simulink model "DrivetrainHevP4"  (R2020a)
settings: Solver=VariableStepAuto  StartTime=0.0  StopTime=inf  RelTol=1e-3  EnableMultiTasking=on
model workspace (MAT data in the model file):
  Aeff = 0.0314159265359
  Af = 2.46
  Bx = 10
  Cd = 0.25
  Cl = 0.1
  Cpm = 0.1
  Cx = 1.65
  Dx = 1
  Ex = 0.01
  FZMAX = 6570
  FZMIN = 0
  Fc = 500
  FsbF = [-700000 -7000 -700 0 700 7000 700000]
  FsbR = [-700000 -7000 -700 0 700 7000 700000]
  FskF = [-8928.57142857 -178.571428571 0 357.142857143 535.714285714 9285.71428571]
  FskR = [-5357.14285714 -107.142857143 0 214.285714286 321.428571429 5571.42857143]
  G = [0 1 2 3 4 5 6]
  G_o = 1
  Iyy = 3000
  Iyy_Whl = 0.8
  J = 0.01
  J1 = 0.01
  J2 = 0.01
  Jd = 0.01
  Ji = 0.2
  Jin = 0.05
  Jin_Cltch = 0.2
  Jin_Cltch2 = 0.01
  Jout = [0.009 0.01 0.01 0.01 0.01 0.01 0.01]
  Jout_Cltch = 0.01
  Jout_Cltch2 = 0.05
  Jt = 0.01
  Jw1 = 0.01
  Jw2 = 0.01
  K_c = 10000
  Lrel = 0.15
  Mass = 1623
  N = [0.001 4.212 2.637 1.8 1.386 1 0.772]
  NF = 2
  NR = 2
  N_P4 = 4.1
  Ndiff = 3.32
  Ndiff_P4 = 4.1
  Ndisk = 1
  Ndisks = 4
  Pabs = 101325
  Press = 7000000
  Re = 0.327
  Reff = 0.11
  Reff_LSD = 0.2
  Rm = 0.15
  T = 300
  Temp_bpts = [313 358]
  Trq_bpts = [25 50 75 100 150 200 250]
  UNLOADED_RADIUS = 0.336
  VXLOW = 2
  aMy = 0.01
  a_CG = 1.09
  alphaMy = 0
  b = Simulink.Parameter
  b.Value = 400
  b.DataType = 'auto'
  b.Dimensions = [1 1]
  b1 = 100
  b1_g = 0.001
  b2 = 100
  b2_g = 0.001
  bMy = 0
  b_CG = 1.7
  b_J = 0.001
  bd = 0.001
  betaMy = 1
  bi = 0.001
  bin = 0.003
  bin_Cltch = 0.003
  bout = [0.003 0.003 0.003 0.003 0.003 0.003 0.003]
  bout_Cltch = 0.003
  br = 0.001
  bt = 0.001
  bw1 = 0.001
  bw2 = 0.001
  cMy = 0
  disk_abore = 0.05
  domega_o = 0
  dw = [0 10 20 40 60 80 100]
  dzdotsF = [-10 -1 -0.1 0 0.1 1 10]
  dzdotsR = [-10 -1 -0.1 0 0.1 1 10]
  dzsF = [-0.005 -0.0001 0 0.2 0.2001 0.2051]
  dzsR = [-0.005 -0.0001 0 0.2 0.2001 0.2051]
  eta = [0.95 0.95 0.95 0.95 0.95 0.95 0.95]
  eta_diff = 0.98
  eta_tbl = [1 1 1 1 1 1 1 1 1 1 1 1 ... (1078 elements, 7x11x7x2)]
  g = 9.81
  h = 0.5
  k = Simulink.Parameter
  k.Value = 10000
  k.DataType = 'auto'
  k.Dimensions = [1 1]
  k1 = 50000
  k2 = 50000
  kappamax = 1.5
  lam_x = 1
  mu_kinetic = 0.35
  mu_static = 0.45
  muc = [0.16 0.13 0.115 0.11 0.105 0.1025 0.10125]
  muk = 0.4
  mus = 0.45
  num_pads = 2
  omega1_c = 3000
  omega2_c = 3000
  omega_bpts = [500.383141081 749.619781963 1002.67614148 1250.9578527 1499.23956393 1747.52127515 1995.80298637 2501.9157054 2998.47912785 4001.15526933 5003.83141081]
  omega_c = Simulink.Parameter
  omega_c.Value = 500
  omega_c.DataType = 'auto'
  omega_c.Dimensions = [1 1]
  omega_o = 0
  omega_o_J = 0
  omegai_o = 0
  omegain_o = 0
  omegal = 94.2477796077
  omegao = 0
  omegaout_o = 0
  omegat_o = 0
  omegau = 83.7758040957
  omegaw1o = 0
  omegaw2o = 0
  phi = [0 0.5 0.6 0.7 0.8 0.87 0.92 0.94 0.96 0.97]
  philu = 0.85
  press = 234400
  psi = [12.2938 12.8588 13.1452 13.6285 14.6163 16.2675 19.3503 22.1046 29.9986 50]
  q_o = 0
  tauC = 0.6
  tauC_1 = 0.1
  tauC_LSD = 0.01
  tauTC = 0.1
  tau_s = 0.08
  tc = 0.01
  theta_o = 0
  theta_o_Veh = 0
  ts = 0.01
  w1_o = 0
  wc = 10
  win_o = 0
  wout_o = 0
  x_o = 0
  xdot_o = 0
  z_o = -0.35
  zdot_o = 0
  zeta = [2.232 1.5462 1.4058 1.2746 1.1528 1.0732 1.0192 0.9983 0.9983 0.9983]
undefined symbols (not defined in the file): Lock, up
libraries: autolibsharedcoupling x4, autolibpowerinfoutils x4, autolibshared x3, autolibshareddiff x2, autolibutils x2, autolibsharedtransfixedgear x1, autolibtrqconv x1
(part 1 of 3)
settings Model: ModifiedByFormat=The MathWorks, Inc.  SimulationMode=accelerator  PauseTimes=10  OrderedModelArguments=off  Creator=The MathWorks, Inc.  LastModifiedBy=The MathWorks, Inc.
settings SolverCC: DecoupledContinuousIntegration=on
settings DataIOCC: DSMLogging=off  ReturnWorkspaceOutputs=off
settings DebuggingCC: MergeDetectMultiDrivingBlocksExec=none  ArithmeticOperatorsInVariantConditions=warning
settings ModelReferenceCC: PropagateSignalLabelsOutOfModel=off
settings SFSimCC: SimUseLocalCustomCode=off
settings RTWCC: RTWUseLocalCustomCode=off
settings CodeAppCC: StateflowObjectComments=on
settings GRTTargetCC: TargetLangStandard=C89/C90 (ANSI)
settings ConfigComp: CovMetricSettings=dsw  CovHtmlReporting=on  CovSaveCumulativeToWorkspaceVar=on  CovSaveSingleToWorkspaceVar=on  CovShowResultsExplorer=off  CovExternalEMLEnable=off
settings SimscapeCC: SimscapeNormalizeSystem=off  SimscapeNominalValues={1, 'bar'; 1, 'cm^3/s'; 1, 'bar*kg/s'; 1, 'kJ/kg'; 1, 'kW'; }

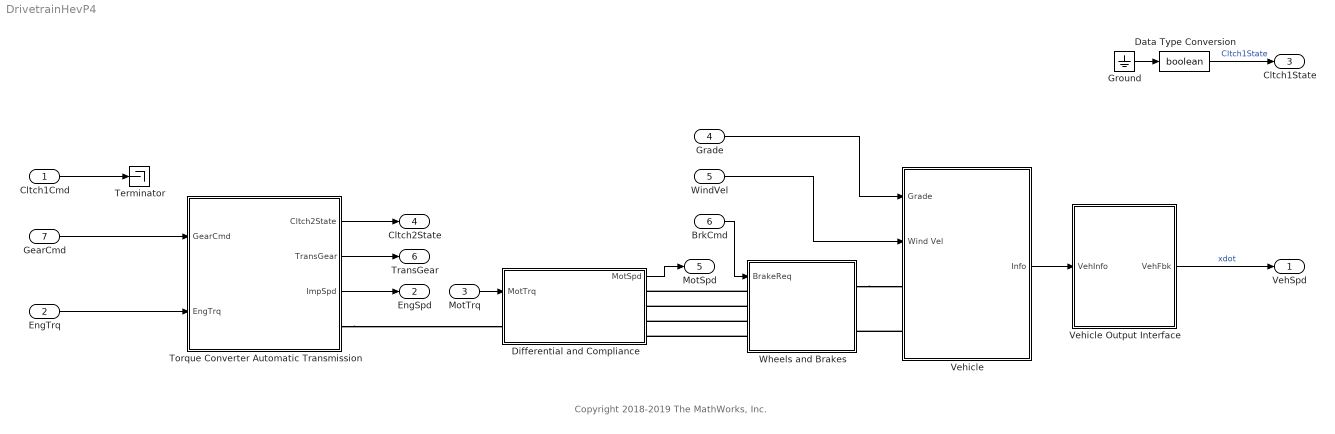
== system DrivetrainHevP4 ==
  note: Copyright 2018-2019 The MathWorks, Inc.
  Cltch1Cmd : Inport
  EngTrq : Inport  Port=2
  MotTrq : Inport  Port=3
  Grade : Inport  Port=4
  WindVel : Inport  Port=5
  BrkCmd : Inport  Port=6
  GearCmd : Inport  Port=7
  Data Type Conversion : DataTypeConversion  OutDataTypeStr=boolean
  Differential and Compliance : Subsystem  VariantControl=2
  Ground : Ground
  Terminator : Terminator
  Torque Converter Automatic Transmission : Subsystem  VariantControl=1
  Vehicle : Subsystem
  Vehicle Output Interface : Subsystem
  Wheels and Brakes : Subsystem  VariantControl=0
  VehSpd : Outport  VectorParamsAs1DForOutWhenUnconnected=off
  EngSpd : Outport  Port=2  VectorParamsAs1DForOutWhenUnconnected=off  BusOutputAsStruct=on
  Cltch1State : Outport  Port=3  VectorParamsAs1DForOutWhenUnconnected=off  BusOutputAsStruct=on
  Cltch2State : Outport  Port=4  VectorParamsAs1DForOutWhenUnconnected=off  BusOutputAsStruct=on
  MotSpd : Outport  Port=5  VectorParamsAs1DForOutWhenUnconnected=off  BusOutputAsStruct=on
  TransGear : Outport  Port=6  VectorParamsAs1DForOutWhenUnconnected=off  BusOutputAsStruct=on
  wires:
  BrkCmd/1 -> Wheels and Brakes/1(BrakeReq)
  Vehicle/1(Info) -> Vehicle Output Interface/1(VehInfo)
  Vehicle Output Interface/1(VehFbk) -> VehSpd/1  "xdot"
  Grade/1 -> Vehicle/1(Grade)
  WindVel/1 -> Vehicle/2(Wind Vel)
  Ground/1 -> Data Type Conversion/1
  Data Type Conversion/1 -> Cltch1State/1  "Cltch1State"
  Torque Converter Automatic Transmission/1(Cltch2State) -> Cltch2State/1
  Torque Converter Automatic Transmission/2(TransGear) -> TransGear/1
  Cltch1Cmd/1 -> Terminator/1
  GearCmd/1 -> Torque Converter Automatic Transmission/1(GearCmd)
  MotTrq/1 -> Differential and Compliance/1(MotTrq)
  EngTrq/1 -> Torque Converter Automatic Transmission/2(EngTrq)
  Torque Converter Automatic Transmission/3(ImpSpd) -> EngSpd/1
  Differential and Compliance/1(MotSpd) -> MotSpd/1
  connections:
  Wheels and Brakes/RConn1 -- Vehicle/LConn1
  Wheels and Brakes/LConn1 -- Differential and Compliance/RConn1
  Wheels and Brakes/LConn3 -- Differential and Compliance/RConn3
  Wheels and Brakes/LConn2 -- Differential and Compliance/RConn2
  Wheels and Brakes/LConn4 -- Differential and Compliance/RConn4
  Vehicle/LConn2 -- Wheels and Brakes/RConn2
  Torque Converter Automatic Transmission/RConn1 -- Differential and Compliance/LConn1

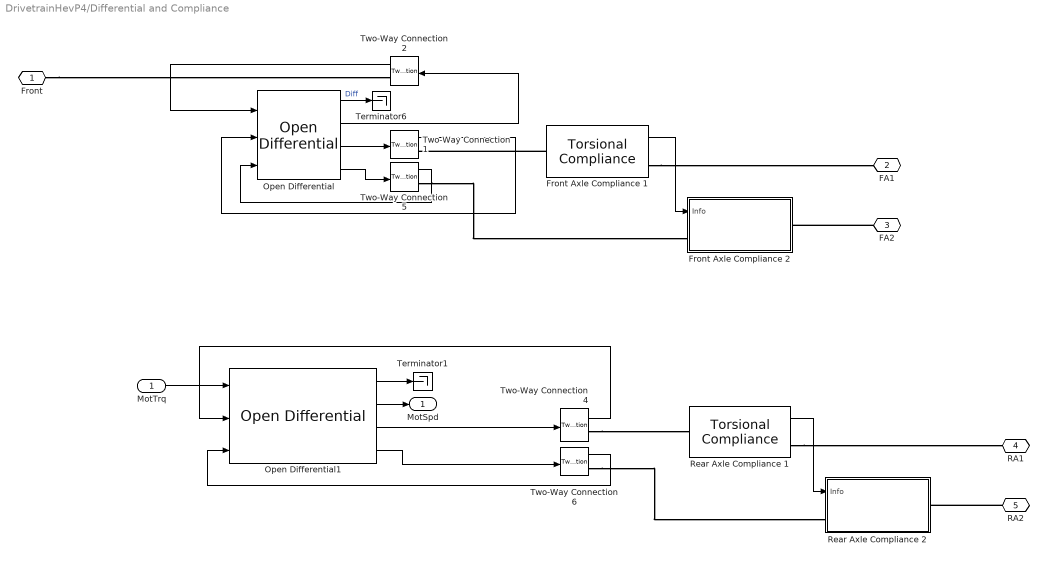
== system DrivetrainHevP4/Differential and Compliance ==
  MotTrq : Inport
  Front Axle Compliance 1 : autolibsharedcoupling/Torsional Compliance  port_config=Two-way connection  extInfo=on  k=k  b=b  theta_o=theta_o  domega_o=domega_o  omega_c=omega_c  blkID=0  aMode=1
      settings: SourceProductBaseCode=PW,MT,VE,VP
  Front Axle Compliance 2 : Subsystem
  Open Differential : autolibshareddiff/Open Differential  DiffEffModelPopup=Constant  InterpMethod=Linear point-slope  extTamb=off  shaftSwitchMask=To the left of center-line  Ndiff=Ndiff  Jd=Jd  bd=bd  Jw1=Jw1  bw1=bw1  Jw2=Jw2  bw2=bw2  omegaw1o=omegaw1o  omegaw2o=omegaw2o  eta=eta_diff  eta_tbl=reshape([0.64 0.76 0.8 0.81 0.83 0.84 0.84 0.56 0.73 0.78 0.8 0.83 0.84 0.84 0.54 0.71 0.77 0.8 0.82 0.84 0.84 0.53 0.71 0.77 0.8 0.83 0.84 0.84 0.51 0.71 0.77 0.8 0.83 0.84 0.85 0.52 0.7 0.77 0.8 0.83 0.84 0.85 0.51 0.71 0.76 0.79 0.83 0.84 0.85 0.5 0.69 0.76 0.79 0.82 0.84 0.85 0.45 0.68 0.75 0.78 0.82 0.84 0.85 0.43 0.67 0.74 0.78 0.81 0.83 0.84 0.38 0.63 0.71 0.75 0.8 0.82 0.83 0.81 0.86 0.88 0.89 0.89 0.89 0.9 0.77 0.85 0.87 0.88 0.89 0.9 0.9 0.72 0.82 0.86 0.87 0.88 0.89 0.9 0.68 0.8 0.84 0.86 0.88 0.89 0.89 0.67 0.8 0.84 0.86 0.88 0.89 0.9 0.67 0.8 0.84 0.86 0.88 0.89 0.9 0.65 0.8 0.84 0.86 0.88 0.89 0.9 0.64 0.79 0.83 0.86 0.88 0.89 0.9 0.63 0.78 0.83 0.86 0.88 0.89 0.9 0.59 0.76 0.82 0.85 0.87 0.89 0.9 0.53 0.73 0.8 0.83 0.86 0.88 0.89], 7, 11, 2)  Trq_bpts=[25, 50, 75, 100, 150, 200, 250]  omega_bpts=[52.4 78.5 105 131 157 183 209 262 314 419 524]  Temp_bpts=[290 358]  Tamb=297.15  maxAbsSpd=5e3  aMode=1
      settings: SourceProductBaseCode=PW,MT,VE,VP
  Open Differential1 : autolibshareddiff/Open Differential  DiffEffModelPopup=Constant  InterpMethod=Linear point-slope  extTamb=off  shaftSwitchMask=To the left of center-line  Ndiff=Ndiff_P4  Jd=Jd  bd=bd  Jw1=Jw1  bw1=bw1  Jw2=Jw2  bw2=bw2  omegaw1o=omegaw1o  omegaw2o=omegaw2o  eta=eta_diff  eta_tbl=reshape([0.64 0.76 0.8 0.81 0.83 0.84 0.84 0.56 0.73 0.78 0.8 0.83 0.84 0.84 0.54 0.71 0.77 0.8 0.82 0.84 0.84 0.53 0.71 0.77 0.8 0.83 0.84 0.84 0.51 0.71 0.77 0.8 0.83 0.84 0.85 0.52 0.7 0.77 0.8 0.83 0.84 0.85 0.51 0.71 0.76 0.79 0.83 0.84 0.85 0.5 0.69 0.76 0.79 0.82 0.84 0.85 0.45 0.68 0.75 0.78 0.82 0.84 0.85 0.43 0.67 0.74 0.78 0.81 0.83 0.84 0.38 0.63 0.71 0.75 0.8 0.82 0.83 0.81 0.86 0.88 0.89 0.89 0.89 0.9 0.77 0.85 0.87 0.88 0.89 0.9 0.9 0.72 0.82 0.86 0.87 0.88 0.89 0.9 0.68 0.8 0.84 0.86 0.88 0.89 0.89 0.67 0.8 0.84 0.86 0.88 0.89 0.9 0.67 0.8 0.84 0.86 0.88 0.89 0.9 0.65 0.8 0.84 0.86 0.88 0.89 0.9 0.64 0.79 0.83 0.86 0.88 0.89 0.9 0.63 0.78 0.83 0.86 0.88 0.89 0.9 0.59 0.76 0.82 0.85 0.87 0.89 0.9 0.53 0.73 0.8 0.83 0.86 0.88 0.89], 7, 11, 2)  Trq_bpts=[25, 50, 75, 100, 150, 200, 250]  omega_bpts=[52.4 78.5 105 131 157 183 209 262 314 419 524]  Temp_bpts=[290 358]  Tamb=297.15  maxAbsSpd=5e3  aMode=1
      settings: SourceProductBaseCode=PW,MT,VE,VP
  Rear Axle Compliance 1 : autolibsharedcoupling/Torsional Compliance  port_config=Two-way connection  extInfo=on  k=k  b=b  theta_o=theta_o  domega_o=domega_o  omega_c=omega_c  blkID=0  aMode=1
      settings: SourceProductBaseCode=PW,MT,VE,VP
  Rear Axle Compliance 2 : Subsystem
  Terminator1 : Terminator
  Terminator6 : Terminator
  Two-Way Connection{1..2,4..6} (5 alike) : TwoWayConnection
  Front : PMIOPort  Side=Left
  FA1 : PMIOPort  Port=2  Side=Right
  FA2 : PMIOPort  Port=3  Side=Right
  RA1 : PMIOPort  Port=4  Side=Right
  RA2 : PMIOPort  Port=5  Side=Right
  MotSpd : Outport  VectorParamsAs1DForOutWhenUnconnected=off
  wires:
  Two-Way Connection6/1 -> Open Differential1/3
  Open Differential1/4 -> Two-Way Connection6/1
  Rear Axle Compliance 1/1 -> Rear Axle Compliance 2/1(Info)
  Two-Way Connection5/1 -> Open Differential/3
  Open Differential/4 -> Two-Way Connection5/1
  Front Axle Compliance 1/1 -> Front Axle Compliance 2/1(Info)
  Two-Way Connection4/1 -> Open Differential1/2
  Open Differential1/3 -> Two-Way Connection4/1
  Open Differential1/1 -> Terminator1/1
  Open Differential/2 -> Two-Way Connection2/1
  Open Differential/3 -> Two-Way Connection1/1
  Two-Way Connection1/1 -> Open Differential/2
  Two-Way Connection2/1 -> Open Differential/1
  Open Differential/1 -> Terminator6/1  "Diff"
  Open Differential1/2 -> MotSpd/1
  MotTrq/1 -> Open Differential1/1
  connections:
  Two-Way Connection6/RConn1 -- Rear Axle Compliance 2/LConn1
  Rear Axle Compliance 1/RConn1 -- RA1/RConn1
  Two-Way Connection4/RConn1 -- Rear Axle Compliance 1/LConn1
  RA2/RConn1 -- Rear Axle Compliance 2/RConn1
  Front Axle Compliance 1/LConn1 -- Two-Way Connection1/RConn1
  Front Axle Compliance 1/RConn1 -- FA1/RConn1
  FA2/RConn1 -- Front Axle Compliance 2/RConn1
  Two-Way Connection5/RConn1 -- Front Axle Compliance 2/LConn1
  Front/RConn1 -- Two-Way Connection2/RConn1

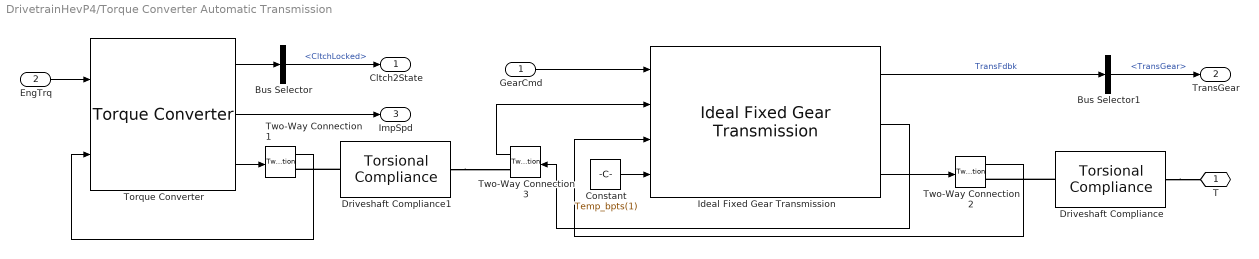
== system DrivetrainHevP4/Torque Converter Automatic Transmission ==
  GearCmd : Inport
  EngTrq : Inport  Port=2
  Bus Selector : BusSelector  OutputSignals=Cltch.CltchLocked
  Bus Selector1 : BusSelector  OutputSignals=Trans.TransGear
  Constant : Constant  Value=Temp_bpts(1)
  Driveshaft Compliance : autolibsharedcoupling/Torsional Compliance  port_config=Two-way connection  extInfo=off  k=k  b=b  theta_o=theta_o  domega_o=domega_o  omega_c=omega_c  blkID=0  aMode=1
      settings: SourceProductBaseCode=PW,MT,VE,VP
  Driveshaft Compliance1 : autolibsharedcoupling/Torsional Compliance  port_config=Two-way connection  extInfo=off  k=k  b=b  theta_o=theta_o  domega_o=domega_o  omega_c=omega_c  blkID=0  aMode=1
      settings: SourceProductBaseCode=PW,MT,VE,VP
  Ideal Fixed Gear Transmission : autolibsharedtransfixedgear/Ideal Fixed Gear Transmission  VariantControl=0  TransEffModelPopup=Gear, input torque, input speed, and temperature  gearInterp=Linear point-slope  G=G  Trq_bpts=Trq_bpts  omega_bpts=omega_bpts  Temp_bpts=Temp_bpts  N=N  Jout=Jout  bout=bout  eta=eta  eta_tbl=eta_tbl  G_o=0  omega_o=omega_o  omegaN_o=0  tau_s=tau_s  maxAbsSpd=5e3  aMode=1
      settings: SourceProductBaseCode=PW,MT,VE,VP
  Torque Converter : autolibtrqconv/Torque Converter  TCType=Lock-up  port_config=Simulink  Ji=Ji  bi=bi  Jt=Jt  bt=bt  omegai_o=omegai_o  omegat_o=omegat_o  phi=phi  KType=Input speed / sqrt(input torque)  psi=psi  zeta=zeta  tauTC=tauTC  InterpMethod=Linear  Reff=Reff  mus=mus  muk=muk  ClutchLocked=off  philu=philu  omegal=omegal  omegau=omegau  K_c=K_c  tauC=tauC  maxAbsSpd=5e3  tau_dl=3000
      settings: AttributesFormatString="Lock-up type:  %<TCType>"  SourceProductBaseCode=PW
  Two-Way Connection1 : TwoWayConnection
  Two-Way Connection2 : TwoWayConnection
  Two-Way Connection3 : TwoWayConnection
  T : PMIOPort  Side=Right
  Cltch2State : Outport  VectorParamsAs1DForOutWhenUnconnected=off
  TransGear : Outport  Port=2  VectorParamsAs1DForOutWhenUnconnected=off
  ImpSpd : Outport  Port=3  VectorParamsAs1DForOutWhenUnconnected=off
  wires:
  Bus Selector1/1 -> TransGear/1  "<TransGear>"
  Constant/1 -> Ideal Fixed Gear Transmission/4
  Bus Selector/1 -> Cltch2State/1  "<CltchLocked>"
  Two-Way Connection3/1 -> Ideal Fixed Gear Transmission/2
  EngTrq/1 -> Torque Converter/1
  Ideal Fixed Gear Transmission/3 -> Two-Way Connection2/1
  Two-Way Connection1/1 -> Torque Converter/2
  Two-Way Connection2/1 -> Ideal Fixed Gear Transmission/3
  Torque Converter/3 -> Two-Way Connection1/1
  Ideal Fixed Gear Transmission/2 -> Two-Way Connection3/1
  Torque Converter/1 -> Bus Selector/1
  Torque Converter/2 -> ImpSpd/1
  Ideal Fixed Gear Transmission/1 -> Bus Selector1/1  "TransFdbk"
  GearCmd/1 -> Ideal Fixed Gear Transmission/1
  connections:
  Driveshaft Compliance/RConn1 -- T/RConn1
  Driveshaft Compliance1/LConn1 -- Two-Way Connection1/RConn1
  Driveshaft Compliance/LConn1 -- Two-Way Connection2/RConn1
  Driveshaft Compliance1/RConn1 -- Two-Way Connection3/RConn1

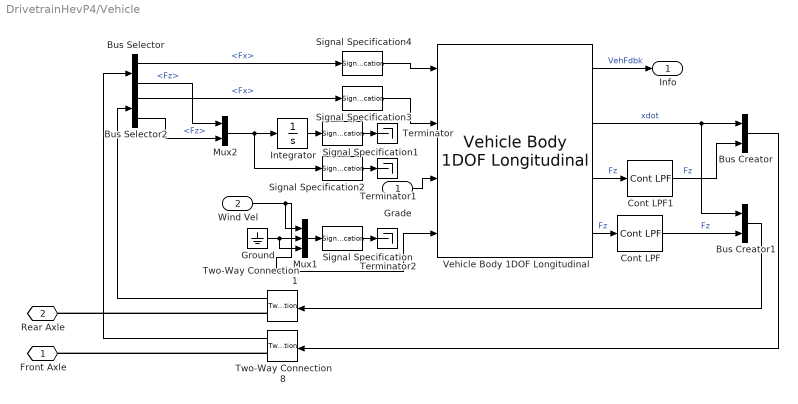
== system DrivetrainHevP4/Vehicle ==
  Grade : Inport  Unit=deg
  Wind Vel : Inport  Port=2  Unit=m/s
  Bus Creator : BusCreator  Inputs=2
  Bus Creator1 : BusCreator  Inputs=2
  Bus Selector : BusSelector  OutputSignals=Fx,Fz
  Bus Selector2 : BusSelector  OutputSignals=Fx,Fz
  Cont LPF : autolibutils/Cont LPF  wc=wc  aMode=aMode
      settings: SourceProductBaseCode=PW,MT,VE,VP
  Cont LPF1 : autolibutils/Cont LPF  wc=wc  aMode=aMode
      settings: SourceProductBaseCode=PW,MT,VE,VP
  Ground : Ground
  Integrator : Integrator
  Mux1 : Mux  Inputs=3
  Mux2 : Mux  Inputs=2
  Signal Specification : SignalSpecification  Unit=m/s
  Signal Specification1 : SignalSpecification  Unit=m
  Signal Specification2 : SignalSpecification  Unit=m/s
  Signal Specification3 : SignalSpecification  Unit=N
  Signal Specification4 : SignalSpecification  Unit=N
  Terminator : Terminator
  Terminator1 : Terminator
  Terminator2 : Terminator
  Two-Way Connection1 : TwoWayConnection
  Two-Way Connection8 : TwoWayConnection
  Vehicle Body 1DOF Longitudinal : autolibshared/Vehicle Body 1DOF Longitudinal  VariantControl=SL  extFMode=off  extMMode=off  extTamb=off  wind3D=off  aMode=1  NF=NF  NR=NR  m=Mass  a=a_CG  b=b_CG  h=h  Cd=Cd  Cl=0  Cpm=0  Af=Af  x_o=x_o  xdot_o=xdot_o  Pabs=Pabs  T=T  g=g
      settings: SourceProductBaseCode=PW,MT,VE,VP
  Front Axle : PMIOPort  Side=Left
  Rear Axle : PMIOPort  Port=2  Side=Left
  Info : Outport  VectorParamsAs1DForOutWhenUnconnected=off
  wires:
  Two-Way Connection1/1 -> Bus Selector2/1
  Bus Selector2/2 -> Mux2/2  "<Fz>"
  Bus Selector2/1 -> Signal Specification3/1  "<Fx>"
  Bus Selector/2 -> Mux2/1  "<Fz>"
  Bus Selector/1 -> Signal Specification4/1  "<Fx>"
  Bus Creator1/1 -> Two-Way Connection1/1
  Bus Creator/1 -> Two-Way Connection8/1
  Signal Specification4/1 -> Vehicle Body 1DOF Longitudinal/1
  Signal Specification3/1 -> Vehicle Body 1DOF Longitudinal/2
  Signal Specification2/1 -> Terminator1/1
  Signal Specification1/1 -> Terminator/1
  Signal Specification/1 -> Terminator2/1
  Grade/1 -> Vehicle Body 1DOF Longitudinal/3
  Wind Vel/1 -> Vehicle Body 1DOF Longitudinal/4, Mux1/1
  Integrator/1 -> Signal Specification1/1
  Mux2/1 -> Signal Specification2/1, Integrator/1
  Vehicle Body 1DOF Longitudinal/4 -> Cont LPF/1  "Fz"
  Mux1/1 -> Signal Specification/1
  Ground/1 -> Mux1/3, Mux1/2
  Vehicle Body 1DOF Longitudinal/1 -> Info/1  "VehFdbk"
  Two-Way Connection8/1 -> Bus Selector/1
  Vehicle Body 1DOF Longitudinal/2 -> Bus Creator/1, Bus Creator1/1  "xdot"
  Vehicle Body 1DOF Longitudinal/3 -> Cont LPF1/1  "Fz"
  Cont LPF/1 -> Bus Creator1/2  "Fz"
  Cont LPF1/1 -> Bus Creator/2  "Fz"
  connections:
  Two-Way Connection1/RConn1 -- Rear Axle/RConn1
  Two-Way Connection8/RConn1 -- Front Axle/RConn1

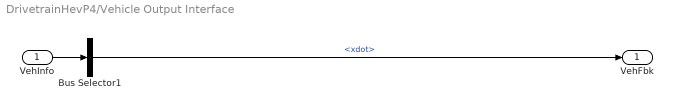
== system DrivetrainHevP4/Vehicle Output Interface ==
  VehInfo : Inport
  Bus Selector1 : BusSelector  OutputSignals=BdyFrm.Cg.Vel.xdot
  VehFbk : Outport  VectorParamsAs1DForOutWhenUnconnected=off
  wires:
  Bus Selector1/1 -> VehFbk/1  "<xdot>"
  VehInfo/1 -> Bus Selector1/1
